simulink model "vipmotion"  (R2020b)
settings: Solver=FixedStepDiscrete  StartTime=0.0  StopTime=inf  RelTol=1e-3
model workspace (MAT data in the model file):
  blockSize = [60 80]
undefined symbols (not defined in the file or in its folder): gray, M, N, sz
libraries: vipmisc x10, dspvision x1, simulink x1, visionanalysis x1
settings Model: FPTRunName=Active  ExtModeAutoUpdateStatusClock=off  Creator=The MathWorks, Inc.  LastModifiedBy=carlo
settings DataIOCC: LimitDataPoints=on  SaveFormat=Array  SaveOutput=off  SaveTime=off  ReturnWorkspaceOutputs=off  SignalLoggingName=sigsOut
settings OptimizationCC: ExpressionDepthLimit=2147483647  InitFltsAndDblsToZero=on  LifeSpan=inf  BufferReusableBoundary=off
settings DebuggingCC: SaveWithParameterizedLinksMsg=none  UnderspecifiedInitializationDetection=Classic  MergeDetectMultiDrivingBlocksExec=none  CheckExecutionContextPreStartOutputMsg=on  CheckExecutionContextRuntimeOutputMsg=on  SignalResolutionControl=TryResolveAllWithWarning  MultiTaskDSMMsg=warning  MultiTaskCondExecSysMsg=none  ParameterPrecisionLossMsg=none  FcnCallInpInsideContextMsg=warning  BusObjectLabelMismatch=none  StateNameClashWarn=warning  SFUnexpectedBacktrackingDiag=warning  SFNoUnconditionalDefaultTransitionDiag=warning  SFExecutionAtInitializationDiag=none  ArithmeticOperatorsInVariantConditions=warning
settings HardwareCC: ProdBitPerPointer=32  ProdBitPerSizeT=32  ProdBitPerPtrDiffT=32  ProdLargestAtomicFloat=None  ProdIntDivRoundTo=Undefined  ProdEndianess=Unspecified  ProdWordSize=32  ProdHWDeviceType=32-bit Generic  TargetBitPerPointer=64  TargetBitPerSizeT=64  TargetBitPerPtrDiffT=64  TargetLongLongMode=on  TargetIntDivRoundTo=Zero  TargetEndianess=LittleEndian  TargetWordSize=64  TargetHWDeviceType=Generic->MATLAB Host Computer  ProdEqTarget=off
settings ModelReferenceCC: PropagateSignalLabelsOutOfModel=off
settings SFSimCC: SimUseLocalCustomCode=off  CustomCodeUndefinedFunction=UseInterfaceOnly
settings RTWCC: RTWUseLocalCustomCode=off
settings CodeAppCC: StateflowObjectComments=on
settings GRTTargetCC: TargetFcnLib=ansi_tfl_tmw.mat  TargetLangStandard=C89/C90 (ANSI)  CombineOutputUpdateFcns=off  GRTInterface=on
settings ConfigComp: CovMetricSettings=dw  CovSaveCumulativeToWorkspaceVar=on  CovSaveSingleToWorkspaceVar=on  CovExternalEMLEnable=off

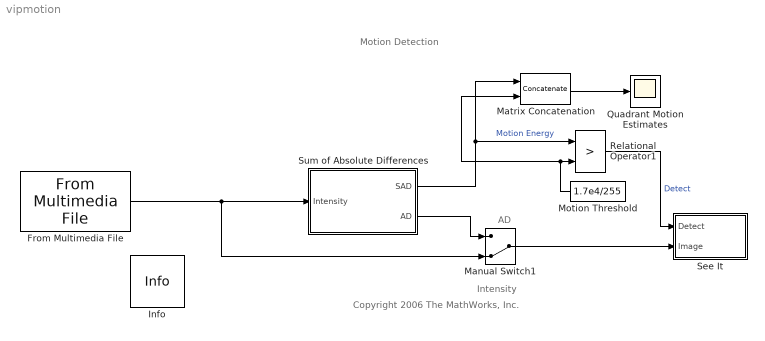
== system vipmotion ==
  note: AD
  note: Motion Detection
  note: Intensity
  note: Copyright 2006 The MathWorks, Inc.
  From Multimedia File : dspvision/From Multimedia File  inputFilename=vipmen.avi  readRange=[1 Inf]  loop=on  numPlays=inf  outputStreams=Video only  videoDataType=single  audioDataType=int16  inheritSampleTime=on  userDefinedSampleTime=1/30  noAudioOutput=off  isIntensityVideo=off  fourcc=Intensity  colorVideoFormat=Separate color signals  outputEOF=off  dataOrg=Column-major  audioFrameSize=1024  computeAudioFrameSize=off  outSamplingMode=Frame based
  Info : vipmisc/Info  SystemSampleTime=-1  VariantActivationTime=update diagram  Latency=0  AutoFrameSizeCalculation=off
      settings: SourceProductBaseCode=VP
  Manual Switch1 : ManualSwitch  CurrentSetting=0
  Matrix Concatenation : Concatenate  Mode=Multidimensional array
  Motion Threshold : Constant  Value=1.7e4/255  VectorParams1D=off  OutDataTypeStr=Inherit: Inherit via back propagation
  Quadrant Motion Estimates : Scope
  Relational Operator1 : RelationalOperator  Operator=>  OutDataTypeStr=boolean  RndMeth=Nearest  InputSameDT=on
  See It : Subsystem
  Sum of Absolute Differences : Subsystem
  wires:
  From Multimedia File/1 -> Sum of Absolute Differences/1(Intensity), Manual Switch1/2
  Sum of Absolute Differences/2(AD) -> Manual Switch1/1
  Sum of Absolute Differences/1(SAD) -> Relational Operator1/1, Matrix Concatenation/1  "Motion Energy"
  Motion Threshold/1 -> Relational Operator1/2, Matrix Concatenation/2
  Manual Switch1/1 -> See It/2(Image)
  Relational Operator1/1 -> See It/1(Detect)  "Detect"
  Matrix Concatenation/1 -> Quadrant Motion Estimates/1

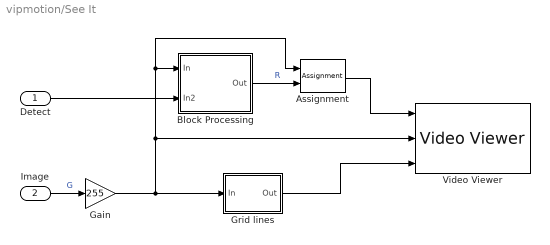
== system vipmotion/See It ==
  Detect : Inport
  Image : Inport  Port=2
  Assignment : Assignment  NumberOfDimensions=2  IndexOptions=Starting index (dialog),Starting index (dialog)  Indices=1,1  OutputSizes=1,1
  Block Processing : Subsystem  DialogController=vipDDGCreate  TreatAsAtomicUnit=on  mask(Block Processing){NumI=2, ParamPort=off, NumO=1, Blocksize={blockSize, [1 1]}, Overlapsize={[0 0]}, Traverse=Row-wise}
      mask prompts: NumI "Number of inputs:"; ParamPort "Add port to supply subsystem parameters"; NumO "Number of outputs:"; Blocksize "Block size:"; Overlapsize "Overlap size:"; Traverse "Order of traversing:"
      mask help:
      | Repeats a user-specified operation on submatrices of the input matrix.
      |
      | This block extracts submatrices of a user-specified size from the input matrix. It sends each submatrix to a subsystem for processing, and then reassembles each subsystem output into the output matrix.
      |
      | Use the Block size and Overlap parameters to specify the size and overlap of each submatrix in cell array format.
      mask init:
      | errmsg = vipblkblockproc(gcbh, NumI, NumO, Blocksize, Overlapsize, Traverse, ParamPort);
      | error(errmsg);
      settings: CopyFcn=set_param(gcb,'LinkStatus','none');
      mask Help: eval('helpview(fullfile(docroot,''toolbox'',''vision'',''vision.map''),''vipblockprocessing'')');
      mask TypeOptions Traverse: Row-wise | Column-wise
      mask Display:
      | disp('Block\n Processing');
      | 
      | if ((NumI == 1) && ParamPort)
      |     port_label('input', 1, 'I');
      | end
      | 
      | if (NumI > 1)
      |     for (i = 1:NumI)
      |         port_label('input', i, ['I' int2str(i)]);
      |     end
      | end
      | 
      | if (ParamPort)
      |     port_label('input', NumI+1, 'P');
      | end
  Gain : Gain  Gain=255  OutDataTypeStr=uint(8)  ParamDataTypeStr=Inherit: Same as input
  Grid lines : Subsystem
  Video Viewer : VideoViewer  imagePorts=separate color signals  colormapValue=gray(256)  FigPos=[753 468 191 153]
  wires:
  Image/1 -> Gain/1  "G"
  Detect/1 -> Block Processing/2(In2)
  Gain/1 -> Assignment/1, Block Processing/1(In), Video Viewer/2, Grid lines/1(In)
  Block Processing/1(Out) -> Assignment/2  "R"
  Assignment/1 -> Video Viewer/1
  Grid lines/1(Out) -> Video Viewer/3

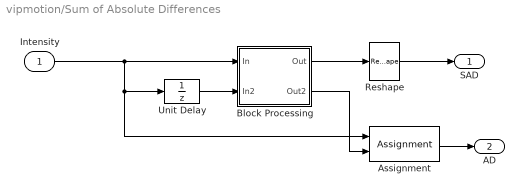
== system vipmotion/Sum of Absolute Differences ==
  Intensity : Inport
  Assignment : Assignment  NumberOfDimensions=2  IndexOptions=Starting index (dialog),Starting index (dialog)  Indices=1,1  OutputSizes=1,1
  Block Processing : Subsystem  DialogController=vipDDGCreate  TreatAsAtomicUnit=on  mask(Block Processing){NumI=2, ParamPort=off, NumO=2, Blocksize={blockSize}, Overlapsize={[0 0]}, Traverse=Row-wise}
      mask prompts: NumI "Number of inputs:"; ParamPort "Add port to supply subsystem parameters"; NumO "Number of outputs:"; Blocksize "Block size:"; Overlapsize "Overlap size:"; Traverse "Order of traversing:"
      mask help:
      | Repeats a user-specified operation on submatrices of the input matrix.
      |
      | This block extracts submatrices of a user-specified size from the input matrix. It sends each submatrix to a subsystem for processing, and then reassembles each subsystem output into the output matrix.
      |
      | Use the Block size and Overlap parameters to specify the size and overlap of each submatrix in cell array format.
      mask init:
      | errmsg = vipblkblockproc(gcbh, NumI, NumO, Blocksize, Overlapsize, Traverse, ParamPort);
      | error(errmsg);
      settings: CopyFcn=set_param(gcb,'LinkStatus','none');
      mask Help: eval('helpview(fullfile(docroot,''toolbox'',''vision'',''vision.map''),''vipblockprocessing'')');
      mask TypeOptions Traverse: Row-wise | Column-wise
      mask Display:
      | disp('Block\n Processing');
      | 
      | if ((NumI == 1) && ParamPort)
      |     port_label('input', 1, 'I');
      | end
      | 
      | if (NumI > 1)
      |     for (i = 1:NumI)
      |         port_label('input', i, ['I' int2str(i)]);
      |     end
      | end
      | 
      | if (ParamPort)
      |     port_label('input', NumI+1, 'P');
      | end
  Reshape : Reshape  OutputDimensionality=Column vector (2-D)  OutputDimensions=[M,N]
  Unit Delay : UnitDelay  SampleTime=-1  HasFrameUpgradeWarning=on
  SAD : Outport  VectorParamsAs1DForOutWhenUnconnected=off
  AD : Outport  Port=2  VectorParamsAs1DForOutWhenUnconnected=off
  wires:
  Unit Delay/1 -> Block Processing/2(In2)
  Block Processing/1(Out) -> Reshape/1
  Reshape/1 -> SAD/1
  Intensity/1 -> Assignment/1, Unit Delay/1, Block Processing/1(In)
  Block Processing/2(Out2) -> Assignment/2
  Assignment/1 -> AD/1

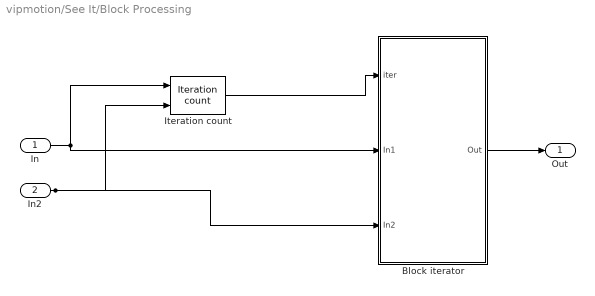
== system vipmotion/See It/Block Processing ==
  In : Inport
  In2 : Inport  Port=2
  Block iterator : Subsystem
      settings: CopyFcn=set_param(gcb,'ReferenceBlock','');
  Iteration count : vipmisc/Iteration count  NumI=NumI  blksize=Blocksize  ovlpsize=Overlapsize
      settings: SourceProductBaseCode=VP
  Out : Outport  VectorParamsAs1DForOutWhenUnconnected=off
  wires:
  Iteration count/1 -> Block iterator/1(iter)
  In/1 -> Iteration count/1, Block iterator/2(In1)
  Block iterator/1(Out) -> Out/1
  In2/1 -> Block iterator/3(In2), Iteration count/2

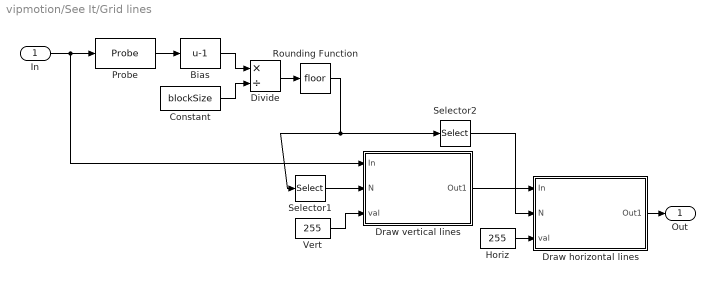
== system vipmotion/See It/Grid lines ==
  In : Inport
  Bias : Bias  Bias=-1
  Constant : Constant  Value=blockSize
  Divide : Product  Inputs=*/
  Draw horizontal lines : Subsystem  TreatAsAtomicUnit=on
  Draw vertical lines : Subsystem  TreatAsAtomicUnit=on
  Horiz : Constant  Value=255  VectorParams1D=off  OutDataTypeStr=Inherit: Inherit via back propagation
  Probe : Probe  ProbeWidth=off  ProbeSampleTime=off  ProbeComplexSignal=off  ProbeSignalDimensions=on
  Rounding Function : Rounding
  Selector1 : Selector  InputPortWidth=2  IndexOptions=Index vector (dialog)  Indices=2  OutputSizes=1
  Selector2 : Selector  InputPortWidth=2  IndexOptions=Index vector (dialog)  Indices=1  OutputSizes=1
  Vert : Constant  Value=255  VectorParams1D=off  OutDataTypeStr=Inherit: Inherit via back propagation
  Out : Outport  VectorParamsAs1DForOutWhenUnconnected=off
  wires:
  In/1 -> Probe/1, Draw vertical lines/1(In)
  Probe/1 -> Bias/1
  Bias/1 -> Divide/1
  Constant/1 -> Divide/2
  Divide/1 -> Rounding Function/1
  Selector1/1 -> Draw vertical lines/2(N)
  Rounding Function/1 -> Selector1/1, Selector2/1
  Vert/1 -> Draw vertical lines/3(val)
  Draw vertical lines/1(Out1) -> Draw horizontal lines/1(In)
  Selector2/1 -> Draw horizontal lines/2(N)
  Horiz/1 -> Draw horizontal lines/3(val)
  Draw horizontal lines/1(Out1) -> Out/1

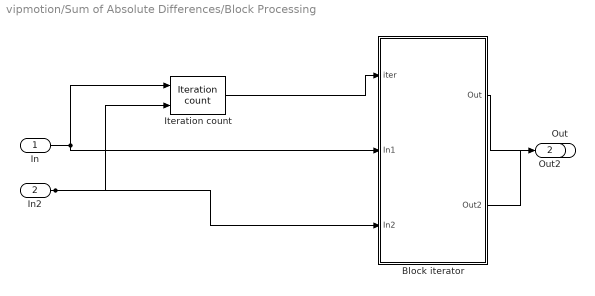
== system vipmotion/Sum of Absolute Differences/Block Processing ==
  In : Inport
  In2 : Inport  Port=2
  Block iterator : Subsystem
      settings: CopyFcn=set_param(gcb,'ReferenceBlock','');
  Iteration count : vipmisc/Iteration count  NumI=NumI  blksize=Blocksize  ovlpsize=Overlapsize
      settings: SourceProductBaseCode=VP
  Out : Outport  VectorParamsAs1DForOutWhenUnconnected=off
  Out2 : Outport  Port=2  VectorParamsAs1DForOutWhenUnconnected=off
  wires:
  Iteration count/1 -> Block iterator/1(iter)
  In/1 -> Iteration count/1, Block iterator/2(In1)
  Block iterator/1(Out) -> Out/1
  In2/1 -> Block iterator/3(In2), Iteration count/2
  Block iterator/2(Out2) -> Out2/1

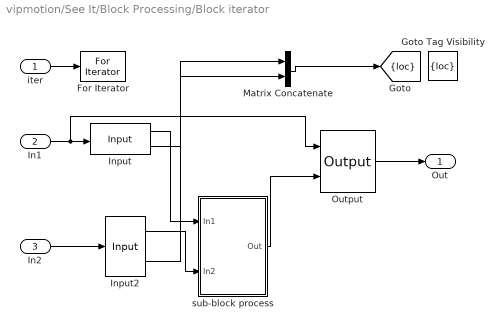
== system vipmotion/See It/Block Processing/Block iterator ==
  iter : Inport
  In1 : Inport  Port=2
  In2 : Inport  Port=3
  For Iterator : ForIterator  IterationSource=external  IterationLimit=(sz(1)/M)*(sz(2)/N)  ShowIterationPort=off  IndexMode=Zero-based  IterationVariableDataType=double
  Goto Tag Visibility : GotoTagVisibility  GotoTag=loc
  Input : vipmisc/Input  Blocksize=Blocksize{1}  Overlapsize=Overlapsize{1}  tverse=Row-wise
      settings: SourceProductBaseCode=VP
  Input2 : vipmisc/Input  Blocksize=Blocksize{2}  Overlapsize=Overlapsize{1}  tverse=Row-wise
      settings: SourceProductBaseCode=VP
  Matrix Concatenate : Concatenate  Mode=Multidimensional array  ConcatenateDimension=2
  Output : vipmisc/Output  Blocksize=Blocksize{1}  Overlapsize=Overlapsize{1}  tverse=Row-wise
      settings: SourceProductBaseCode=VP
  sub-block process : Subsystem
  Out : Outport  VectorParamsAs1DForOutWhenUnconnected=off
  tag scope: loc=scoped
  wires:
  Matrix Concatenate/1 -> [loc]
  Input/2 -> Matrix Concatenate/1
  Input/1 -> sub-block process/1(In1)
  iter/1 -> For Iterator/1
  In1/1 -> Input/1, Output/1
  Output/1 -> Out/1
  sub-block process/1(Out) -> Output/2
  Input2/2 -> Matrix Concatenate/2
  In2/1 -> Input2/1
  Input2/1 -> sub-block process/2(In2)

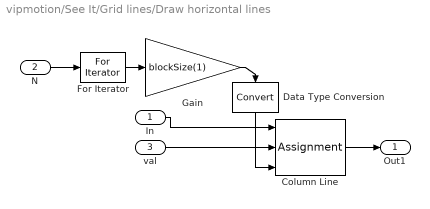
== system vipmotion/See It/Grid lines/Draw horizontal lines ==
  In : Inport
  N : Inport  Port=2
  val : Inport  Port=3
  Column Line : Assignment  NumberOfDimensions=2  IndexOptions=Index vector (port),Assign all  Indices=60,-1  OutputSizes=1,1
  Data Type Conversion : DataTypeConversion
  For Iterator : ForIterator  IterationSource=external
  Gain : Gain  Gain=blockSize(1)
  Out1 : Outport  VectorParamsAs1DForOutWhenUnconnected=off
  wires:
  Data Type Conversion/1 -> Column Line/3
  Gain/1 -> Data Type Conversion/1
  val/1 -> Column Line/2
  In/1 -> Column Line/1
  Column Line/1 -> Out1/1
  For Iterator/1 -> Gain/1
  N/1 -> For Iterator/1

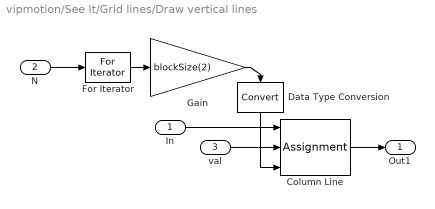
== system vipmotion/See It/Grid lines/Draw vertical lines ==
  In : Inport
  N : Inport  Port=2
  val : Inport  Port=3
  Column Line : Assignment  NumberOfDimensions=2  IndexOptions=Assign all,Index vector (port)  Indices=60,-1  OutputSizes=1,1
  Data Type Conversion : DataTypeConversion
  For Iterator : ForIterator  IterationSource=external
  Gain : Gain  Gain=blockSize(2)
  Out1 : Outport  VectorParamsAs1DForOutWhenUnconnected=off
  wires:
  N/1 -> For Iterator/1
  For Iterator/1 -> Gain/1
  Column Line/1 -> Out1/1
  In/1 -> Column Line/1
  val/1 -> Column Line/2
  Gain/1 -> Data Type Conversion/1
  Data Type Conversion/1 -> Column Line/3

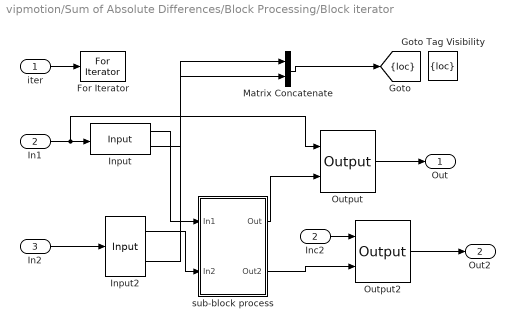
== system vipmotion/Sum of Absolute Differences/Block Processing/Block iterator ==
  iter : Inport
  In1 : Inport  Port=2
  In2 : Inport  Port=3
  For Iterator : ForIterator  IterationSource=external  IterationLimit=(sz(1)/M)*(sz(2)/N)  ShowIterationPort=off  IndexMode=Zero-based  IterationVariableDataType=double
  Goto Tag Visibility : GotoTagVisibility  GotoTag=loc
  Inc2 : InportShadow  Port=2
  Input : vipmisc/Input  Blocksize=Blocksize{1}  Overlapsize=Overlapsize{1}  tverse=Row-wise
      settings: SourceProductBaseCode=VP
  Input2 : vipmisc/Input  Blocksize=Blocksize{1}  Overlapsize=Overlapsize{1}  tverse=Row-wise
      settings: SourceProductBaseCode=VP
  Matrix Concatenate : Concatenate  Mode=Multidimensional array  ConcatenateDimension=2
  Output : vipmisc/Output  Blocksize=Blocksize{1}  Overlapsize=Overlapsize{1}  tverse=Row-wise
      settings: SourceProductBaseCode=VP
  Output2 : vipmisc/Output  Blocksize=Blocksize{1}  Overlapsize=Overlapsize{1}  tverse=Row-wise
      settings: SourceProductBaseCode=VP
  sub-block process : Subsystem
  Out : Outport  VectorParamsAs1DForOutWhenUnconnected=off
  Out2 : Outport  Port=2  VectorParamsAs1DForOutWhenUnconnected=off
  tag scope: loc=scoped
  wires:
  Matrix Concatenate/1 -> [loc]
  Input/2 -> Matrix Concatenate/1
  Input/1 -> sub-block process/1(In1)
  iter/1 -> For Iterator/1
  In1/1 -> Input/1, Output/1
  Output/1 -> Out/1
  sub-block process/1(Out) -> Output/2
  Input2/2 -> Matrix Concatenate/2
  In2/1 -> Input2/1
  Input2/1 -> sub-block process/2(In2)
  Inc2/1 -> Output2/1
  Output2/1 -> Out2/1
  sub-block process/2(Out2) -> Output2/2

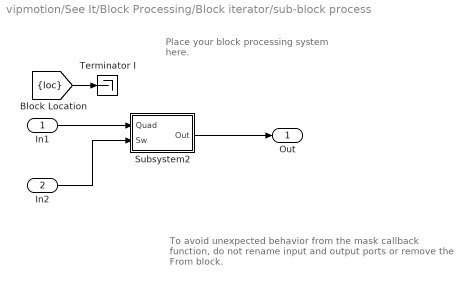
== system vipmotion/See It/Block Processing/Block iterator/sub-block process ==
  note: To avoid unexpected behavior from the mask
      | callback function, do not rename input and output ports or
      | remove the From block.
  note: Place your block
      | processing system here.
  In1 : Inport
  In2 : Inport  Port=2
  Subsystem2 : Subsystem
  Terminator I : Terminator
  Out : Outport  VectorParamsAs1DForOutWhenUnconnected=off
  wires:
  [loc] -> Terminator I/1
  In2/1 -> Subsystem2/2(Sw)
  Subsystem2/1(Out) -> Out/1
  In1/1 -> Subsystem2/1(Quad)

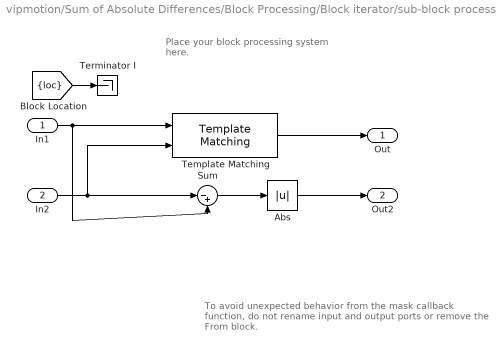
== system vipmotion/Sum of Absolute Differences/Block Processing/Block iterator/sub-block process ==
  note: To avoid unexpected behavior from the mask
      | callback function, do not rename input and output ports or
      | remove the From block.
  note: Place your block
      | processing system here.
  In1 : Inport
  In2 : Inport  Port=2
  Abs : Abs  SaturateOnIntegerOverflow=on
  Sum : Sum  Inputs=|-+
  Template Matching : visionanalysis/Template Matching  metric=Sum of absolute differences  output=Metric matrix  method=Exhaustive  nMetric=off  nSize=3  roi=off  roiValid=off  roundingMode=Floor  overflowMode=off  prodOutputMode=Binary point scaling  prodOutputWordLength=32  prodOutputFracLength=0  accumMode=Binary point scaling  accumWordLength=32  accumFracLength=0
      settings: SourceProductBaseCode=VP
  Terminator I : Terminator
  Out : Outport  VectorParamsAs1DForOutWhenUnconnected=off
  Out2 : Outport  Port=2  VectorParamsAs1DForOutWhenUnconnected=off
  wires:
  [loc] -> Terminator I/1
  Template Matching/1 -> Out/1
  Abs/1 -> Out2/1
  Sum/1 -> Abs/1
  In2/1 -> Sum/1, Template Matching/2
  In1/1 -> Sum/2, Template Matching/1

== system vipmotion/See It/Block Processing/Block iterator/sub-block process/Subsystem2 ==
  Quad : Inport
  Sw : Inport  Port=2
  Bitwise Logical Operator : simulink/Logic and Bit Operations/Bitwise Operator  logicop=XOR  UseBitMask=on  BitMask='FF'  BitMaskRealWorld=Stored Integer
  Switch : Switch  Criteria=u2 ~= 0  SaturateOnIntegerOverflow=on  InputSameDT=on
  Out : Outport  VectorParamsAs1DForOutWhenUnconnected=off
  wires:
  Quad/1 -> Switch/3, Bitwise Logical Operator/1
  Bitwise Logical Operator/1 -> Switch/1
  Sw/1 -> Switch/2
  Switch/1 -> Out/1
